simulink model "ESD Lamp Simulink Model"  (R2023b)
settings: Solver=VariableStepAuto  StartTime=0.0  StopTime=100  RelTol=1e-3
libraries: commrandsrc3 x1
(part 2 of 2)

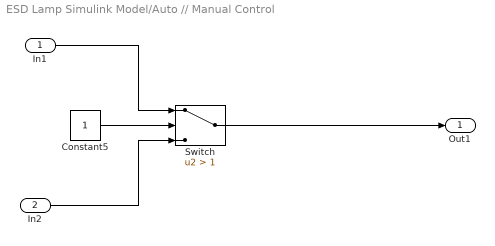
== system ESD Lamp Simulink Model/Auto // Manual Control ==
  In1 : Inport
  In2 : Inport  Port=2
  Constant5 : Constant
  Switch : Switch  Criteria=u2 > Threshold  Threshold=1  SaturateOnIntegerOverflow=off  InputSameDT=off
  Out1 : Outport
  wires:
  In2/1 -> Switch/3
  Constant5/1 -> Switch/2
  Switch/1 -> Out1/1
  In1/1 -> Switch/1

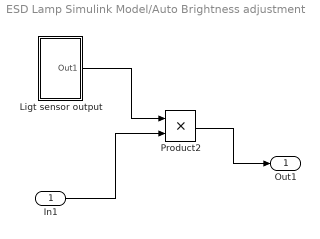
== system ESD Lamp Simulink Model/Auto Brightness adjustment ==
  In1 : Inport
  Ligt sensor output : Subsystem
  Product2 : Product
  Out1 : Outport
  wires:
  Ligt sensor output/1(Out1) -> Product2/1
  Product2/1 -> Out1/1
  In1/1 -> Product2/2

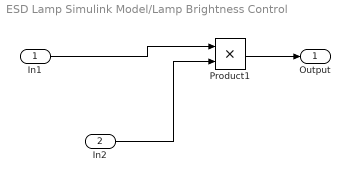
== system ESD Lamp Simulink Model/Lamp Brightness Control ==
  In1 : Inport
  In2 : Inport  Port=2
  Product1 : Product
  Output : Outport
  wires:
  Product1/1 -> Output/1
  In1/1 -> Product1/1
  In2/1 -> Product1/2

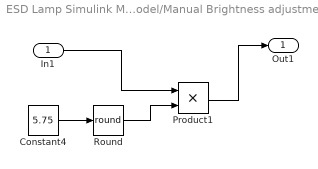
== system ESD Lamp Simulink Model/Manual Brightness adjustment ==
  In1 : Inport
  Constant4 : Constant  Value=5.75
  Product1 : Product
  Round : Rounding  Operator=round
  Out1 : Outport
  wires:
  Round/1 -> Product1/2
  Constant4/1 -> Round/1
  Product1/1 -> Out1/1
  In1/1 -> Product1/1

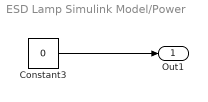
== system ESD Lamp Simulink Model/Power  ==
  Constant3 : Constant  Value=0
  Out1 : Outport
  wires:
  Constant3/1 -> Out1/1

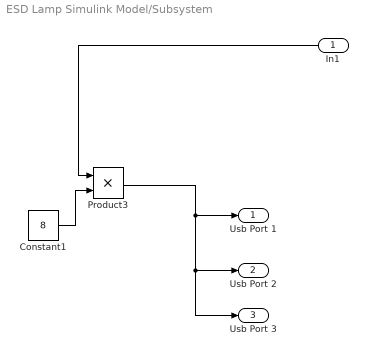
== system ESD Lamp Simulink Model/Subsystem ==
  In1 : Inport
  Constant1 : Constant  Value=8
  Product3 : Product
  Usb Port 1 : Outport
  Usb Port 2 : Outport  Port=2
  Usb Port 3 : Outport  Port=3
  wires:
  Product3/1 -> Usb Port 3/1, Usb Port 2/1, Usb Port 1/1
  Constant1/1 -> Product3/2
  In1/1 -> Product3/1

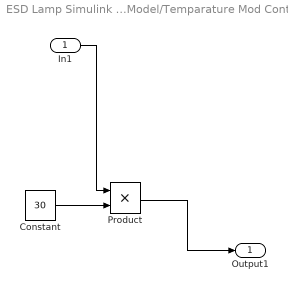
== system ESD Lamp Simulink Model/Temparature Mod Control ==
  In1 : Inport
  Constant : Constant  Value=30
  Product : Product
  Output1 : Outport
  wires:
  Constant/1 -> Product/2
  Product/1 -> Output1/1
  In1/1 -> Product/1

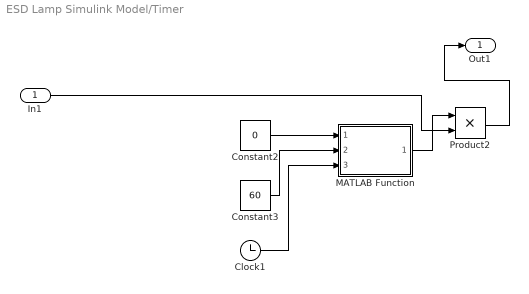
== system ESD Lamp Simulink Model/Timer ==
  In1 : Inport
  Clock1 : Clock
  Constant2 : Constant  Value=0
  Constant3 : Constant  Value=60
  MATLAB Function : MATLAB Function  TreatAsAtomicUnit=on
  Product2 : Product
  Out1 : Outport
  wires:
  MATLAB Function/1(timerOutput) -> Product2/1
  Clock1/1 -> MATLAB Function/3(simTime)
  In1/1 -> Product2/2
  Product2/1 -> Out1/1
  Constant2/1 -> MATLAB Function/1(timerEnable)
  Constant3/1 -> MATLAB Function/2(timeInput)

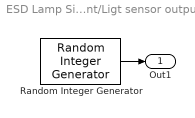
== system ESD Lamp Simulink Model/Auto Brightness adjustment/Ligt sensor output ==
  Random Integer Generator : commrandsrc3/Random Integer Generator  SetSize=8  SeedSource=Auto  Seed=0  SampleTime=5  SamplesPerFrame=1  OutputDataType=double  SimulateUsing=Interpreted execution
  Out1 : Outport
  wires:
  Random Integer Generator/1 -> Out1/1

== matlab function ESD Lamp Simulink Model/Timer/MATLAB Function ==
  data: timerEnable input; timerOutput output; timeInput input; simTime input
function timerOutput = timerControl(timerEnable, timeInput, simTime)
    
    persistent startTime lastTimeInput

    if isempty(startTime)
        startTime = 0;       % initial start time
    end
    if isempty(lastTimeInput)
        lastTimeInput = timeInput;  % store last input duration
    end

    
    timerOutput = 1;

    if timerEnable == 0
        % Timer OFF
        timerOutput = 1;
        startTime = 0;       % reset start time
        lastTimeInput = timeInput; % keep track of input change
    else
        % Timer ON
        
        if startTime == 0 || lastTimeInput ~= timeInput
            startTime = simTime;   % reset start time
            lastTimeInput = timeInput; 
        end

     
        elapsed = simTime - startTime;
        if elapsed >= timeInput
            timerOutput = 0; 
        else
            timerOutput = 1; 
        end
    end
end
